simulink model "Hierarcical_controller_temp_with_estim"  (R2022b)
settings: Solver=VariableStepAuto  StartTime=0.0  StopTime=120  RelTol=1e-3
InitFcn:
  | %% INITIALIZATION
  | 
  | %% UAV PARAMETERS
  | 
  | mass = 2;
  | Ib = diag([1.2416 1.2416 2*1.2416]);
  | g = 9.81;
  | e3=[0 0 1]';
  | Tf=120;
  | %% SAMPLING TIME
  | Ts=0.001;
  | 
  | %%
  | %data for Simulink
  | pos_0 = [x0 y0 z0];
  | lin_vel_0 = [dot_x0 dot_y0 dot_z0];
  | w_bb_0 = [0 0 0];
  | eta_b_0 = [0 0 0];
  | eta_b_dot_0 = [0 0 0];
  | %% momentum based estimator param
  | b=40;
  | 
  | r=2; %order of the estimator
  | 
  | 
  | 
  | s=tf('s');
  | G=b^r/(b+s)^r;
  | 
  | c=cell2mat(G.Denominator);
  | 
  | c=c(2:end);
  | 
  | K=zeros(length(r));
  | 
  | P=1; %product of the gains K_i
  | for i=1:r
  |     K(i)=c(i)/P;
  |     P=P*K(i);
  | end
  | K=flip(K);
values from neighbouring files (symbols this model uses):
  dot_x0 = 0    [poly7.m]
  dot_y0 = 0    [poly7.m]
  dot_z0 = 0    [poly7.m]
  i = find(Nodes==Open(1,end))    [DFS.m]
  Track_path = DFS(A_adj,2,path)    [BRRT_3D.m]    (also in GOOD_PATH.mat = [3 15.8545082605 15.9232549014 27.6290043449 38.9996108348 4)
  x0 = pi(1)    [poly7.m]
  y0 = pi(2)    [poly7.m]
  z0 = pi(3)    [poly7.m]
libraries: robotcorelib x1, uavutilslib x1
settings Model: Creator=fabioruggiero  LastModifiedBy=storm
settings ModelReferenceCC: EnableRefExpFcnMdlSchedulingChecks=on

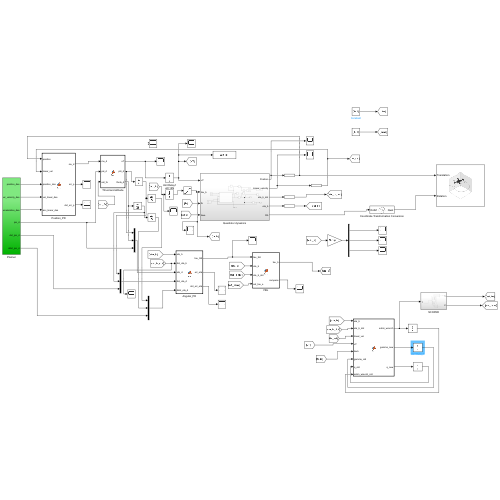
[thumbnail: Simulink's stored preview of the top-level diagram]
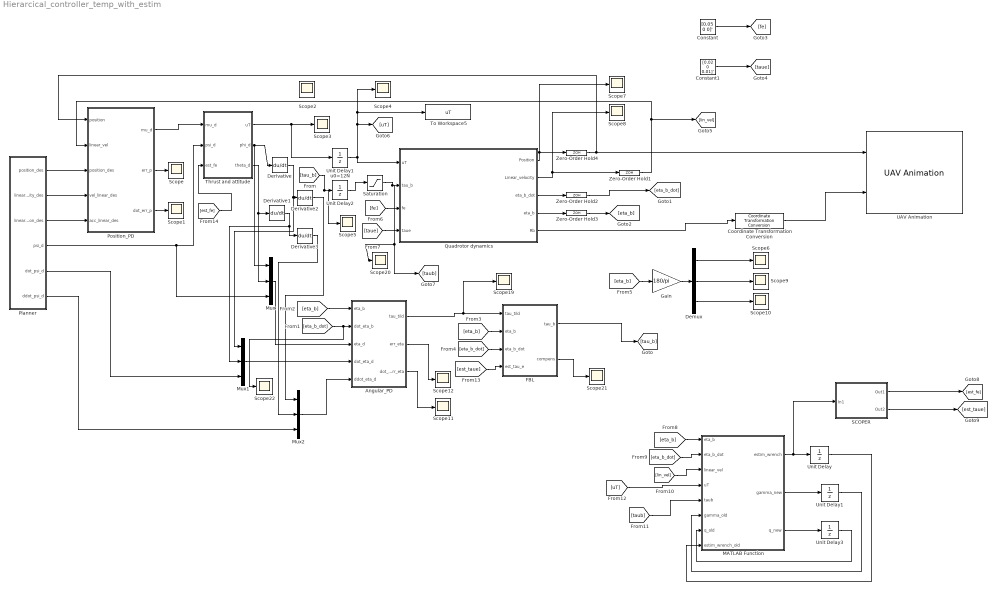
== system Hierarcical_controller_temp_with_estim ==
  Angular_PD : MATLAB Function  TreatAsAtomicUnit=on
  Constant : Constant  Value=[0.05 0 0]'
  Constant1 : Constant  Value=[0.02 0 0.01]'
  Coordinate Transformation Conversion : robotcorelib/Coordinate Transformation Conversion  InputRepresentation=Rotation Matrix  InputEulerSequence=ZYX  ShowTrVecInputPort=on  OutputRepresentation=Quaternion  OutputEulerSequence=XYZ  ShowTrVecOutputPort=on  SimulateUsing=Interpreted execution
  Demux : Demux  Outputs=3
  Derivative{,1..3} (4 alike) : Derivative
  FBL : MATLAB Function  TreatAsAtomicUnit=on
  Gain : Gain  Gain=180/pi
  MATLAB Function : MATLAB Function  TreatAsAtomicUnit=on
  Mux : Mux  Inputs=3
  Mux1 : Mux  Inputs=3
  Mux2 : Mux  Inputs=3
  Planner : Subsystem
  Position_PD : MATLAB Function  TreatAsAtomicUnit=on
  Quadrotor dynamics : Subsystem
  SCOPER : Subsystem
  Saturation : Saturate  UpperLimit=0.8  LowerLimit=-0.8
  Scope{,1..12,19..22} (17 alike) : Scope
  Thrust and attitude : MATLAB Function  TreatAsAtomicUnit=on
  To Workspace5 : ToWorkspace  VariableName=uT  SaveFormat=Structure With Time  SampleTime=-1
  UAV Animation : uavutilslib/UAV Animation  UAVType=Multirotor  UAVSize=1  InertialZDirection=Down  SampleTime=0.01
  Unit Delay : UnitDelay  InitialCondition=zeros(6,1)  SampleTime=Ts  HasFrameUpgradeWarning=on
  Unit Delay1 : UnitDelay  InitialCondition=zeros(6,r)  SampleTime=Ts  HasFrameUpgradeWarning=on
  Unit Delay1 u0=12N : UnitDelay  InitialCondition=mass*9.81  SampleTime=Ts
  Unit Delay2 : UnitDelay  InitialCondition=[0 0 0]  SampleTime=Ts
  Unit Delay3 : UnitDelay  InitialCondition=zeros(6,1)  SampleTime=Ts  HasFrameUpgradeWarning=on
  Zero-Order Hold{1..4} (4 alike) : ZeroOrderHold  SampleTime=Ts
  wires:
  Planner/2(linear_velocity_des) -> Position_PD/4(vel_linear_des)
  Planner/1(position_des) -> Position_PD/3(position_des)
  Quadrotor dynamics/2(Linear_velocity) -> Scope8/1, Zero-Order Hold1/1
  Quadrotor dynamics/1(Position) -> Scope7/1, Zero-Order Hold4/1
  Coordinate Transformation Conversion/1 -> UAV Animation/2
  Position_PD/3(dot_err_p) -> Scope1/1
  Position_PD/2(err_p) -> Scope/1
  Planner/3(linear_acceleration_des) -> Position_PD/5(acc_linear_des)
  Unit Delay1 u0=12N/1 -> Quadrotor dynamics/1(uT), [uT], Scope4/1, To Workspace5/1
  Zero-Order Hold1/1 -> [lin_vel], Position_PD/2(linear_vel)
  Position_PD/1(mu_d) -> Thrust and attitude/1(mu_d)
  Thrust and attitude/1(uT) -> Unit Delay1 u0=12N/1, Scope3/1
  Planner/4(psi_d) -> Mux/3, Thrust and attitude/2(psi_d)
  Thrust and attitude/2(phi_d) -> Mux/1, Derivative/1
  Thrust and attitude/3(theta_d) -> Mux/2, Derivative1/1
  Derivative/1 -> Mux1/1, Derivative2/1
  Derivative1/1 -> Mux1/2, Derivative3/1
  Mux/1 -> Angular_PD/3(eta_d)
  Planner/5(dot_psi_d) -> Mux1/3
  Mux1/1 -> Angular_PD/4(dot_eta_d)
  Derivative2/1 -> Mux2/1
  Derivative3/1 -> Mux2/2
  Planner/6(ddot_psi_d) -> Mux2/3
  Mux2/1 -> Angular_PD/5(ddot_eta_d)
  [tau_b] -> Scope5/1, Unit Delay2/1
  Quadrotor dynamics/3(eta_b_dot) -> Zero-Order Hold2/1
  Quadrotor dynamics/4(eta_b) -> Zero-Order Hold3/1
  Zero-Order Hold2/1 -> [eta_b_dot]
  [eta_b_dot] -> Scope22/1, Angular_PD/2(dot_eta_b)
  Zero-Order Hold3/1 -> [eta_b]
  [eta_b] -> Angular_PD/1(eta_b)
  [eta_b] -> FBL/2(eta_b)
  [eta_b_dot] -> FBL/3(eta_b_dot)
  [eta_b] -> Gain/1
  Demux/1 -> Scope6/1
  Demux/2 -> Scope9/1
  Demux/3 -> Scope10/1
  Gain/1 -> Demux/1
  Angular_PD/2(err_eta) -> Scope12/1
  Angular_PD/3(dot_err_eta) -> Scope11/1
  Zero-Order Hold4/1 -> UAV Animation/1, Position_PD/1(position)
  Quadrotor dynamics/5(Rb) -> Coordinate Transformation Conversion/1
  Constant/1 -> [fe]
  Constant1/1 -> [taue]
  [taue] -> Quadrotor dynamics/4(taue)
  [fe] -> Quadrotor dynamics/3(fe)
  MATLAB Function/3(q_new) -> Unit Delay3/1
  Unit Delay3/1 -> MATLAB Function/7(q_old)
  MATLAB Function/2(gamma_new) -> Unit Delay1/1
  Unit Delay1/1 -> MATLAB Function/6(gamma_old)
  MATLAB Function/1(estim_wrench) -> SCOPER/1(In1), Unit Delay/1
  Unit Delay/1 -> MATLAB Function/8(estim_wrench_old)
  [eta_b] -> MATLAB Function/1(eta_b)
  [eta_b_dot] -> MATLAB Function/2(eta_b_dot)
  [lin_vel] -> MATLAB Function/3(linear_vel)
  [taub] -> MATLAB Function/5(taub)
  [uT] -> MATLAB Function/4(uT)
  [est_taue] -> FBL/4(est_tau_e)
  [est_fe] -> Thrust and attitude/3(est_fe)
  Unit Delay2/1 -> Saturation/1
  FBL/2(compens) -> Scope21/1
  Angular_PD/1(tau_tild) -> FBL/1(tau_tild), Scope19/1
  FBL/1(tau_b) -> [tau_b]
  Saturation/1 -> Scope20/1, [taub], Quadrotor dynamics/2(tau_b)
  SCOPER/1(Out1) -> [est_fe]
  SCOPER/2(Out2) -> [est_taue]

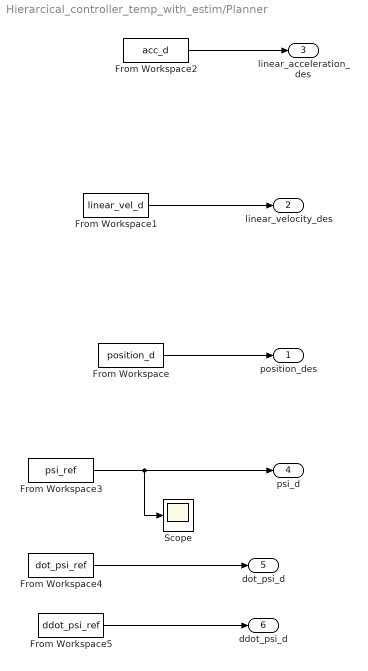
== system Hierarcical_controller_temp_with_estim/Planner ==
  From Workspace : FromWorkspace  VariableName=position_d
  From Workspace1 : FromWorkspace  VariableName=linear_vel_d
  From Workspace2 : FromWorkspace  VariableName=acc_d
  From Workspace3 : FromWorkspace  VariableName=psi_ref
  From Workspace4 : FromWorkspace  VariableName=dot_psi_ref
  From Workspace5 : FromWorkspace  VariableName=ddot_psi_ref
  Scope : Scope
  position_des : Outport
  linear_velocity_des : Outport  Port=2
  linear_acceleration_des : Outport  Port=3
  psi_d : Outport  Port=4
  dot_psi_d : Outport  Port=5
  ddot_psi_d : Outport  Port=6
  wires:
  From Workspace/1 -> position_des/1
  From Workspace1/1 -> linear_velocity_des/1
  From Workspace2/1 -> linear_acceleration_des/1
  From Workspace3/1 -> Scope/1, psi_d/1
  From Workspace4/1 -> dot_psi_d/1
  From Workspace5/1 -> ddot_psi_d/1

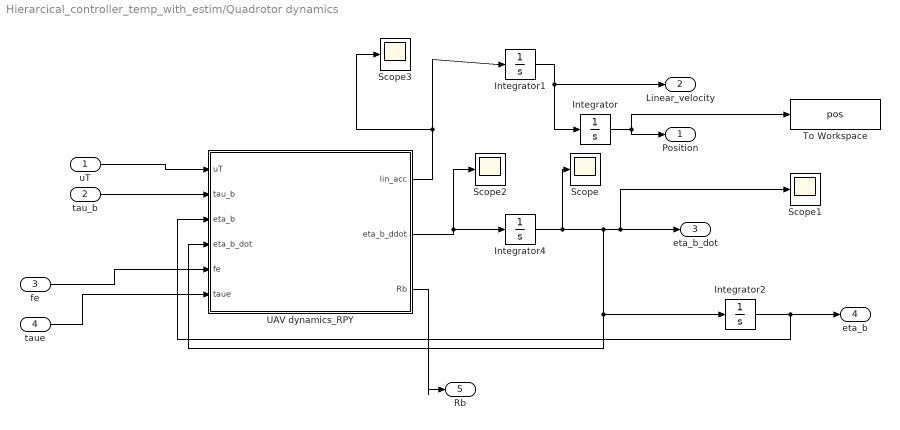
== system Hierarcical_controller_temp_with_estim/Quadrotor dynamics ==
  uT : Inport
  tau_b : Inport  Port=2
  fe : Inport  Port=3
  taue : Inport  Port=4
  Integrator : Integrator  InitialCondition=Track_path(1,:)
  Integrator1 : Integrator  InitialCondition=lin_vel_0
  Integrator2 : Integrator  InitialCondition=eta_b_0
  Integrator4 : Integrator  InitialCondition=eta_b_dot_0
  Scope{,1..3} (4 alike) : Scope
  To Workspace : ToWorkspace  VariableName=pos  SaveFormat=Structure With Time  SampleTime=-1
  UAV dynamics_RPY : MATLAB Function  TreatAsAtomicUnit=on
  Position : Outport
  Linear_velocity : Outport  Port=2
  eta_b_dot : Outport  Port=3
  eta_b : Outport  Port=4
  Rb : Outport  Port=5
  wires:
  tau_b/1 -> UAV dynamics_RPY/2(tau_b)
  UAV dynamics_RPY/1(lin_acc) -> Scope3/1, Integrator1/1
  uT/1 -> UAV dynamics_RPY/1(uT)
  Integrator1/1 -> Integrator/1, Linear_velocity/1
  Integrator/1 -> Position/1, To Workspace/1
  Integrator4/1 -> Scope/1, UAV dynamics_RPY/4(eta_b_dot), Integrator2/1, Scope1/1, eta_b_dot/1
  Integrator2/1 -> UAV dynamics_RPY/3(eta_b), eta_b/1
  UAV dynamics_RPY/3(Rb) -> Rb/1
  UAV dynamics_RPY/2(eta_b_ddot) -> Integrator4/1, Scope2/1
  fe/1 -> UAV dynamics_RPY/5(fe)
  taue/1 -> UAV dynamics_RPY/6(taue)

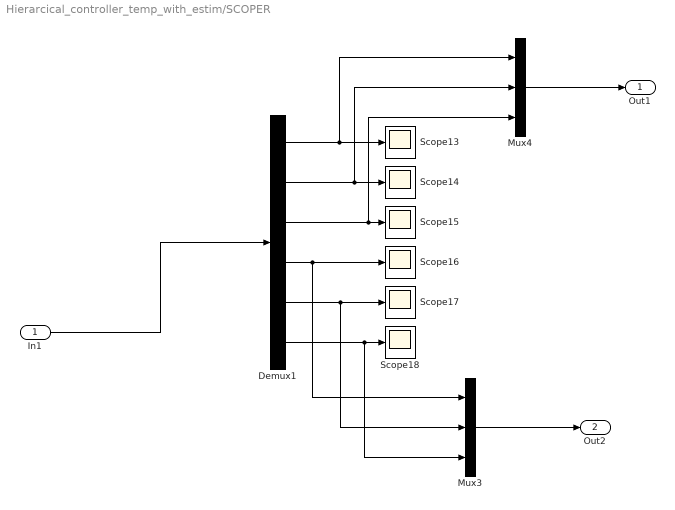
== system Hierarcical_controller_temp_with_estim/SCOPER ==
  In1 : Inport
  Demux1 : Demux  Outputs=6
  Mux3 : Mux  Inputs=3
  Mux4 : Mux  Inputs=3
  Scope{13..18} (6 alike) : Scope
  Out1 : Outport
  Out2 : Outport  Port=2
  wires:
  In1/1 -> Demux1/1
  Mux4/1 -> Out1/1
  Demux1/3 -> Mux4/3, Scope15/1
  Demux1/5 -> Mux3/2, Scope17/1
  Demux1/2 -> Mux4/2, Scope14/1
  Demux1/1 -> Mux4/1, Scope13/1
  Demux1/4 -> Mux3/1, Scope16/1
  Demux1/6 -> Mux3/3, Scope18/1
  Mux3/1 -> Out2/1

== matlab function Hierarcical_controller_temp_with_estim/MATLAB Function ==
  data: eta_b input; estim_wrench output; eta_b_dot input; linear_vel input; uT input; taub input; gamma_new output; q_new output; gamma_old input; q_old input; estim_wrench_old input; mass parameter; Ib parameter; r parameter; K parameter; Ts parameter; g parameter; e3 parameter
function [estim_wrench, gamma_new, q_new] = fcn(eta_b,eta_b_dot,linear_vel,uT,taub,gamma_old,q_old,estim_wrench_old, mass, Ib,r, K,Ts,g, e3)
    
    
    
    q_new=[mass*eye(3) zeros(3,3);zeros(3,3) M_fun(eta_b,Ib)]*[linear_vel;eta_b_dot];
    C=C_fun(eta_b,eta_b_dot,Ib);
    Q=Q_fun(eta_b);
    Rb=R_fun(eta_b);
    gamma_new=gamma_old;
    gamma_new(:,1)=gamma_old(:,1)+K(1)*((q_new-q_old)-Ts*[mass*g*e3-uT*Rb*e3;C'*eta_b_dot+Q'*taub]-Ts*estim_wrench_old);
    
    if r>=2
        for i=2:r
            
            gamma_new(:,i)=gamma_old(:,i)+Ts*K(i)*(-estim_wrench_old+gamma_old(:,i-1));

        end
        
    end
    estim_wrench=gamma_new(:,r);



end




function S=skew(w)

if(numel(w)~= 1)

S= [0 -w(3) w(2);
w(3) 0 -w(1);
-w(2) w(1) 0];

else

S= zeros(3);

end

end

function Q_dot=Q_dot_fun(eta_b,eta_b_dot)

 
Q_dot=[0 0 -cos(eta_b(2))*eta_b_dot(2);

0 -sin(eta_b(1))*eta_b_dot(1) -sin(eta_b(2))*sin(eta_b(1))*eta_b_dot(2)+cos(eta_b(2))*cos(eta_b(1))*eta_b_dot(1);

0 -cos(eta_b(1))*eta_b_dot(1) -sin(eta_b(2))*cos(eta_b(1))*eta_b_dot(2)-cos(eta_b(2))*sin(eta_b(1))*eta_b_dot(1)];

end



function M=M_fun(eta_b,Ib)

Q=Q_fun(eta_b);

M=Q'*Ib*Q;


end


function C=C_fun(eta_b,eta_b_dot,Ib)

Q=Q_fun(eta_b);
S=skew(Q*eta_b_dot);
Q_dot=Q_dot_fun(eta_b,eta_b_dot);
C=Q'*S*Ib*Q+Q'*Ib*Q_dot;


end

function Q = Q_fun(RPY)
Q=[1 0 -sin(RPY(2));
    0 cos(RPY(1)) cos(RPY(2))*sin(RPY(1))
    0 -sin(RPY(1)) cos(RPY(1))*cos(RPY(2))];
end

function Rb = R_fun(eta_b)
Rb=[cos(eta_b(2))*cos(eta_b(3)) sin(eta_b(1))*sin(eta_b(2))*cos(eta_b(3))-cos(eta_b(1))*sin(eta_b(3)) cos(eta_b(1))*sin(eta_b(2))*cos(eta_b(3))+sin(eta_b(1))*sin(eta_b(3));
    cos(eta_b(2))*sin(eta_b(3)) sin(eta_b(1))*sin(eta_b(2))*sin(eta_b(3))+cos(eta_b(1))*cos(eta_b(3)) cos(eta_b(1))*sin(eta_b(2))*sin(eta_b(3))-sin(eta_b(1))*cos(eta_b(3));
-sin(eta_b(2)) sin(eta_b(1))*cos(eta_b(2)) cos(eta_b(1))*cos(eta_b(2))];
end

== matlab function Hierarcical_controller_temp_with_estim/Position_PD ==
  data: position input; mu_d output; linear_vel input; position_des input; vel_linear_des input; acc_linear_des input; err_p output; dot_err_p output
function [mu_d, err_p, dot_err_p] = fcn(position, linear_vel,position_des, vel_linear_des, acc_linear_des)

Kp=[20*eye(3) 20*eye(3)];
err_p=position-position_des;
dot_err_p=linear_vel-vel_linear_des;

mu_d=-Kp*[err_p;dot_err_p]+acc_linear_des;

end

== matlab function Hierarcical_controller_temp_with_estim/Thrust and attitude ==
  data: mu_d input; uT output; psi_d input; phi_d output; theta_d output; mass parameter size=1; est_fe input
function [uT, phi_d, theta_d] = fcn(mu_d,psi_d,mass,est_fe)

g=9.81;

mu_sign=mu_d-1/mass*est_fe;

uT=mass*sqrt(mu_sign(1)^2+mu_sign(2)^2+(mu_sign(3)-g)^2);

phi_d=asin((mass/uT)*(mu_sign(2)*cos(psi_d)-mu_sign(1)*sin(psi_d)));

theta_d=atan((mu_sign(1)*cos(psi_d)+mu_sign(2)*sin(psi_d))/(mu_sign(3)-g));

end

== matlab function Hierarcical_controller_temp_with_estim/Angular_PD ==
  data: eta_b input; tau_tild output; dot_eta_b input; eta_d input; dot_eta_d input; ddot_eta_d input; err_eta output; dot_err_eta output
function [tau_tild ,err_eta, dot_err_eta] = fcn(eta_b,dot_eta_b,eta_d,dot_eta_d,ddot_eta_d)

Ke=[30*eye(3) 30*eye(3)];
err_eta=eta_b-eta_d;
dot_err_eta=dot_eta_b-dot_eta_d;

tau_tild=-Ke*[err_eta;dot_err_eta]+ddot_eta_d;




end

== matlab function Hierarcical_controller_temp_with_estim/FBL ==
  data: tau_tild input; tau_b output size=3; eta_b input; eta_b_dot input; Ib parameter; est_tau_e input; compens output
function [tau_b, compens] = fcn(tau_tild,eta_b,eta_b_dot,Ib,est_tau_e)


Q=Q_fun(eta_b);
C=C_fun(eta_b,eta_b_dot,Ib);


compens=inv(Q)'*est_tau_e;

tau_b= Ib*Q*tau_tild + inv(Q)'*C*eta_b_dot-inv(Q)'*est_tau_e;
end


function S=skew(w)

if(numel(w)~= 1)

S= [0 -w(3) w(2);
w(3) 0 -w(1);
-w(2) w(1) 0];

else

S= zeros(3);

end

end



function Q = Q_fun(RPY)
Q=[1 0 -sin(RPY(2));
    0 cos(RPY(1)) cos(RPY(2))*sin(RPY(1))
    0 -sin(RPY(1)) cos(RPY(1))*cos(RPY(2))];
end

function Q_dot=Q_dot_fun(eta_b,eta_b_dot)

 
Q_dot=[0 0 -cos(eta_b(2))*eta_b_dot(2);

0 -sin(eta_b(1))*eta_b_dot(1) -sin(eta_b(2))*sin(eta_b(1))*eta_b_dot(2)+cos(eta_b(2))*cos(eta_b(1))*eta_b_dot(1);

0 -cos(eta_b(1))*eta_b_dot(1) -sin(eta_b(2))*cos(eta_b(1))*eta_b_dot(2)-cos(eta_b(2))*sin(eta_b(1))*eta_b_dot(1)];

end





function C=C_fun(eta_b,eta_b_dot,Ib)
Q=Q_fun(eta_b);
S=skew(Q*eta_b_dot);
Q_dot=Q_dot_fun(eta_b,eta_b_dot);
C=Q'*S*Ib*Q+Q'*Ib*Q_dot;
end

== matlab function Hierarcical_controller_temp_with_estim/Quadrotor dynamics/UAV dynamics_RPY ==
  data: uT input size=1; tau_b input size=3; lin_acc output size=3; eta_b input size=3; eta_b_dot input; mass parameter size=1; Ib parameter size=[3,3]; eta_b_ddot output size=3; Rb output; fe input; taue input
function [lin_acc,eta_b_ddot,Rb] = fcn(uT,tau_b,eta_b,eta_b_dot,mass, Ib,fe,taue)

M=M_fun(eta_b,Ib);
C=C_fun(eta_b,eta_b_dot,Ib);
Q=Q_fun(eta_b);
Rb=R_fun(eta_b);

lin_acc = 9.81*[0 0 1]'-(uT/mass)*Rb*[0 0 1]'+fe/mass;


eta_b_ddot=inv(M)*(-C*eta_b_dot+Q'*tau_b+taue);


end

function S=skew(w)

if(numel(w)~= 1)

S= [0 -w(3) w(2);
w(3) 0 -w(1);
-w(2) w(1) 0];

else

S= zeros(3);

end

end

function Q_dot=Q_dot_fun(eta_b,eta_b_dot)

 
Q_dot=[0 0 -cos(eta_b(2))*eta_b_dot(2);

0 -sin(eta_b(1))*eta_b_dot(1) -sin(eta_b(2))*sin(eta_b(1))*eta_b_dot(2)+cos(eta_b(2))*cos(eta_b(1))*eta_b_dot(1);

0 -cos(eta_b(1))*eta_b_dot(1) -sin(eta_b(2))*cos(eta_b(1))*eta_b_dot(2)-cos(eta_b(2))*sin(eta_b(1))*eta_b_dot(1)];

end



function M=M_fun(eta_b,Ib)

Q=Q_fun(eta_b);

M=Q'*Ib*Q;


end


function C=C_fun(eta_b,eta_b_dot,Ib)

Q=Q_fun(eta_b);
S=skew(Q*eta_b_dot);
Q_dot=Q_dot_fun(eta_b,eta_b_dot);
C=Q'*S*Ib*Q+Q'*Ib*Q_dot;


end

function Q = Q_fun(RPY)
Q=[1 0 -sin(RPY(2));
    0 cos(RPY(1)) cos(RPY(2))*sin(RPY(1))
    0 -sin(RPY(1)) cos(RPY(1))*cos(RPY(2))];
end

function Rb = R_fun(eta_b)
Rb=[cos(eta_b(2))*cos(eta_b(3)) sin(eta_b(1))*sin(eta_b(2))*cos(eta_b(3))-cos(eta_b(1))*sin(eta_b(3)) cos(eta_b(1))*sin(eta_b(2))*cos(eta_b(3))+sin(eta_b(1))*sin(eta_b(3));
    cos(eta_b(2))*sin(eta_b(3)) sin(eta_b(1))*sin(eta_b(2))*sin(eta_b(3))+cos(eta_b(1))*cos(eta_b(3)) cos(eta_b(1))*sin(eta_b(2))*sin(eta_b(3))-sin(eta_b(1))*cos(eta_b(3));
-sin(eta_b(2)) sin(eta_b(1))*cos(eta_b(2)) cos(eta_b(1))*cos(eta_b(2))];
end
